simulink model "MPC_mobile_base"  (R2018b)
settings: Solver=ode4  StartTime=0.0  StopTime=60  FixedStep=T  RelTol=1e-3
values from neighbouring files (symbols this model uses):
  N = 3    [MPC_dyn_N=3arc traj.mat]    (also in MPC_dyn_N=3arc traj_active.mat; MPC_dyn_N=3complex traj.mat; MPC_dyn_N=3complex traj_active.mat; MPC_dyn_N=6arc traj.mat = 6)
  T = 0.5    [MPC_dyn_N=3arc traj.mat]    (also in MPC_dyn_N=3arc traj_active.mat; MPC_dyn_N=3complex traj.mat; MPC_dyn_N=3complex traj_active.mat; MPC_dyn_N=6arc traj.mat)
  xd = [0 0 0 0 0 0.000654498469498 0.0758636207458 4.96526307585e-05 0.00261799387799 0.227590374774 0.000446873251435 0.00589048622548 ... (153 elements, 3x51)]    [MPC_dyn_N=3arc traj.mat]    (also in MPC_dyn_N=3arc traj_active.mat; MPC_dyn_N=3complex traj.mat = [0 0 0 0.25 0 0 0.5 0 2.44929359829e-17 0.75 -0.024302237621; MPC_dyn_N=3complex traj_active.mat = [0 0 0 0.25 0 0 0.5 0 2.44929359829e-17 0.75 -0.024302237621; MPC_dyn_N=6arc traj.mat)
undefined symbols (not defined in the file or in its folder): DiscIntNeverNeededParam
libraries: simulink x3, templibrary x1
settings Model: Creator=RaffaelePC  LastModifiedBy=Francesco Gennari
settings DebuggingCC: UnderSpecifiedDimensionMsg=warning

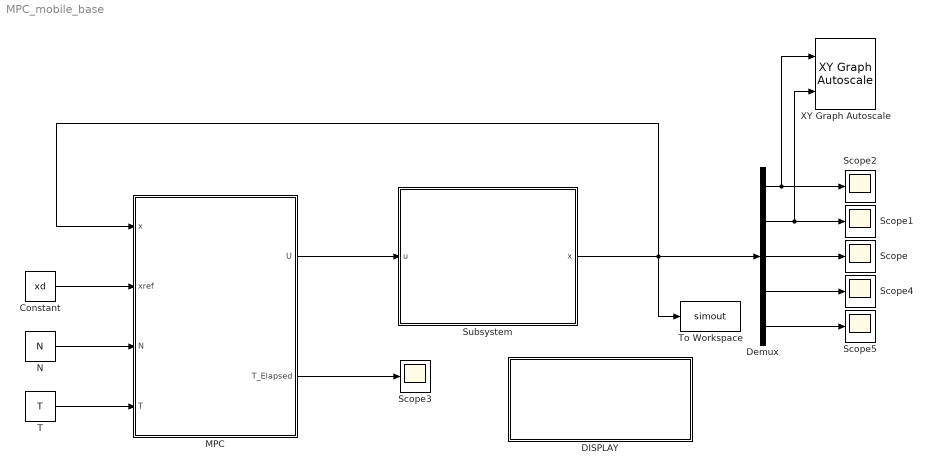
== system MPC_mobile_base ==
  Constant : Constant  Value=xd
  DISPLAY : Subsystem
  Demux : Demux  Outputs=5
  MPC : Subsystem
      mask Display: fprintf('MPC CONTROLLER')
  N : Constant  Value=N
  Scope{,1..5} (6 alike) : Scope
  Subsystem : Subsystem
      mask Display: disp('{\bf\fontsize{10}DYNAMIC SYSTEM}', 'texmode','on');
  T : Constant  Value=T
  To Workspace : ToWorkspace  VariableName=simout  SaveFormat=Timeseries  SampleTime=-1
  XY Graph Autoscale : templibrary/XY Graph  Autoscale  xmin=-1  xmax=1  ymin=-1  ymax=1  st=-1
  wires:
  MPC/1(U) -> Subsystem/1(u)
  N/1 -> MPC/3(N)
  T/1 -> MPC/4(T)
  Constant/1 -> MPC/2(xref)
  Subsystem/1(x) -> To Workspace/1, MPC/1(x), Demux/1
  Demux/3 -> Scope/1
  Demux/1 -> XY Graph Autoscale/1, Scope2/1
  Demux/2 -> XY Graph Autoscale/2, Scope1/1
  MPC/2(T_Elapsed) -> Scope3/1
  Demux/5 -> Scope5/1
  Demux/4 -> Scope4/1

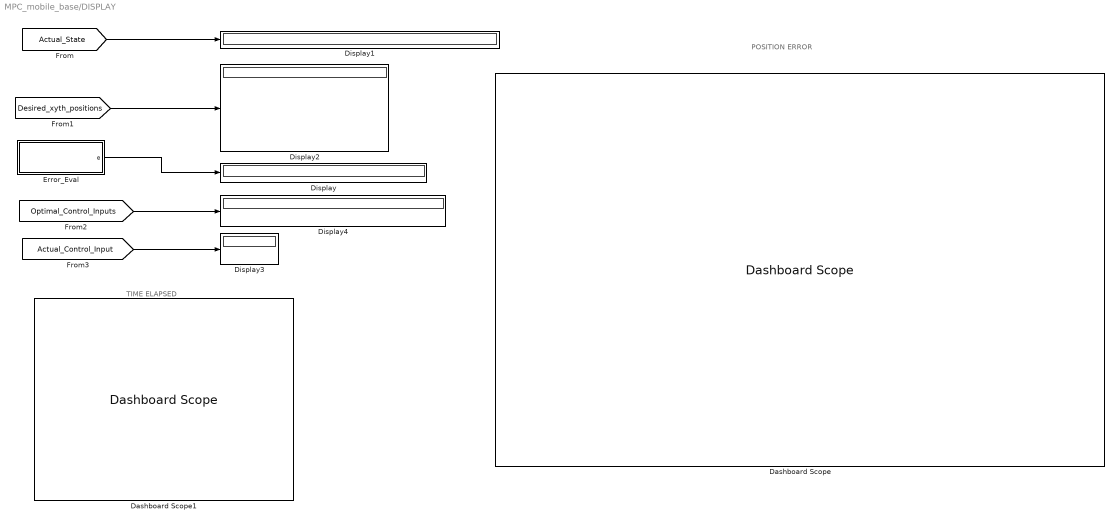
== system MPC_mobile_base/DISPLAY ==
  note: POSITION ERROR
  note: TIME ELAPSED
  Dashboard Scope : DashboardScope  WebBlockId=507  Ymin=-0.5  Ymax=0.5
  Dashboard Scope1 : DashboardScope  WebBlockId=516  Ymin=0  Ymax=1
  Display{,1..4} (5 alike) : Display
  "Error_Eval " : Subsystem
  wires:
  [Optimal_Control_Inputs] -> Display4/1
  [Desired_xyth_positions] -> Display2/1
  [Actual_Control_Input] -> Display3/1
  [Actual_State] -> Display1/1
  "Error_Eval "/1(e) -> Display/1

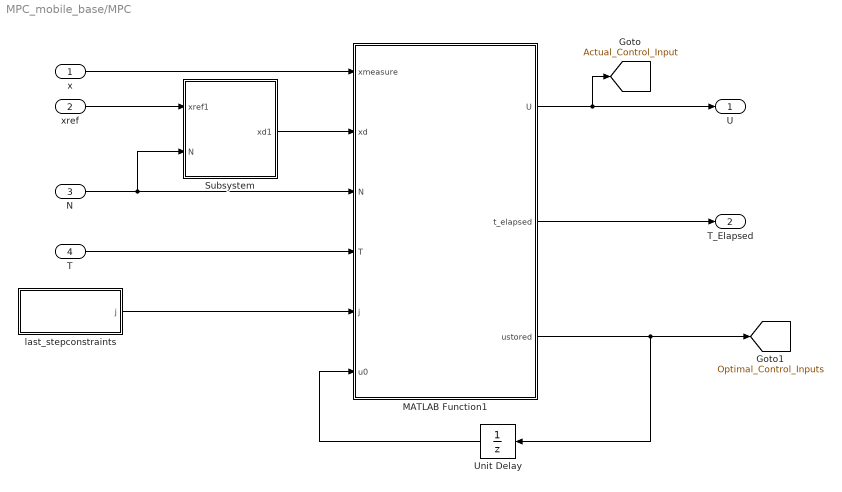
== system MPC_mobile_base/MPC ==
  x : Inport
  xref : Inport  Port=2
  N : Inport  Port=3
  T : Inport  Port=4
  MATLAB Function1 : MATLAB Function  TreatAsAtomicUnit=on
  Subsystem : Subsystem
  Unit Delay : UnitDelay  InitialCondition=zeros(2,N)  SampleTime=-1
  last_stepconstraints : Subsystem
  U : Outport
  T_Elapsed : Outport  Port=2
  tag scope: Actual_Control_Input=global, Optimal_Control_Inputs=global
  wires:
  Subsystem/1(xd1) -> MATLAB Function1/2(xd)
  MATLAB Function1/1(U) -> [Actual_Control_Input], U/1
  MATLAB Function1/3(ustored) -> Unit Delay/1, [Optimal_Control_Inputs]
  Unit Delay/1 -> MATLAB Function1/6(u0)
  xref/1 -> Subsystem/1(xref1)
  x/1 -> MATLAB Function1/1(xmeasure)
  N/1 -> Subsystem/2(N), MATLAB Function1/3(N)
  T/1 -> MATLAB Function1/4(T)
  last_stepconstraints/1(j) -> MATLAB Function1/5(j)
  MATLAB Function1/2(t_elapsed) -> T_Elapsed/1

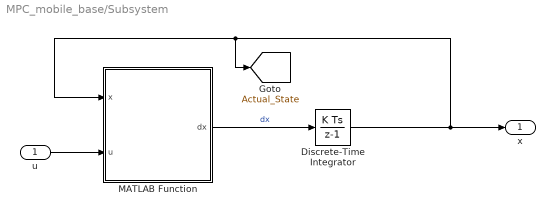
== system MPC_mobile_base/Subsystem ==
  u : Inport
  Discrete-Time Integrator : DiscreteIntegrator  InitialCondition=[xd(:,1).' 0 0]'  SampleTime=-1  ICPrevOutput=DiscIntNeverNeededParam  ICPrevScaledInput=DiscIntNeverNeededParam
  MATLAB Function : MATLAB Function  TreatAsAtomicUnit=on
  x : Outport
  tag scope: Actual_State=global
  wires:
  u/1 -> MATLAB Function/2(u)
  MATLAB Function/1(dx) -> Discrete-Time Integrator/1  "dx"
  Discrete-Time Integrator/1 -> [Actual_State], MATLAB Function/1(x), x/1

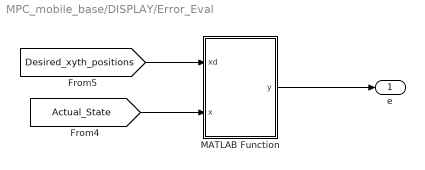
== system MPC_mobile_base/DISPLAY/Error_Eval  ==
  MATLAB Function : MATLAB Function  TreatAsAtomicUnit=on
  e : Outport
  wires:
  MATLAB Function/1(y) -> e/1
  [Desired_xyth_positions] -> MATLAB Function/1(xd)
  [Actual_State] -> MATLAB Function/2(x)

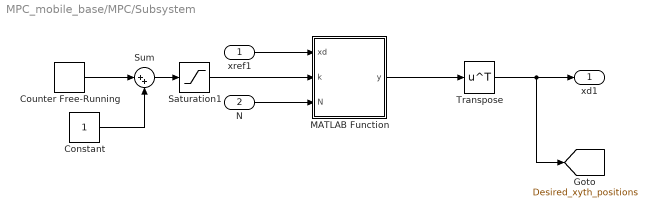
== system MPC_mobile_base/MPC/Subsystem ==
  xref1 : Inport
  N : Inport  Port=2
  Constant : Constant
  Counter Free-Running : simulink/Sources/Counter Free-Running  NumBits=12  tsamp=-1
  MATLAB Function : MATLAB Function  TreatAsAtomicUnit=on
  Saturation1 : Saturate  UpperLimit=size(xd,2)
  Sum : Sum  Inputs=|++
  Transpose : Math  Operator=transpose  SaturateOnIntegerOverflow=on
  xd1 : Outport
  tag scope: Desired_xyth_positions=global
  wires:
  Transpose/1 -> [Desired_xyth_positions], xd1/1
  MATLAB Function/1(y) -> Transpose/1
  N/1 -> MATLAB Function/3(N)
  xref1/1 -> MATLAB Function/1(xd)
  Constant/1 -> Sum/2
  Counter Free-Running/1 -> Sum/1
  Sum/1 -> Saturation1/1
  Saturation1/1 -> MATLAB Function/2(k)

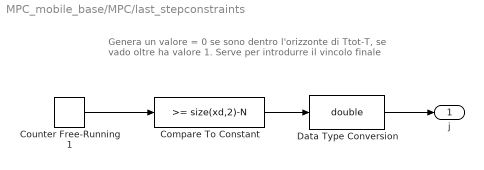
== system MPC_mobile_base/MPC/last_stepconstraints ==
  note: Genera un valore = 0 se sono dentro l'orizzonte di Ttot-T, se vado oltre ha valore 1. Serve per introdurre il vincolo finale
  Compare To Constant : simulink/Logic and Bit Operations/Compare To Constant  relop=>=  const=size(xd,2)-N  OutDataTypeStr=boolean
  Counter Free-Running1 : simulink/Sources/Counter Free-Running  NumBits=12  tsamp=-1
  Data Type Conversion : DataTypeConversion  OutDataTypeStr=double
  j : Outport
  wires:
  Compare To Constant/1 -> Data Type Conversion/1
  Counter Free-Running1/1 -> Compare To Constant/1
  Data Type Conversion/1 -> j/1

== matlab function MPC_mobile_base/MPC/Subsystem/MATLAB Function ==
  settings: updateMethod=DISCRETE  sampleTime=T
  data: xd input; y output size=[3 N+1]; k input; N input
function y  = fcn(xd,k,N)

if size(xd,2)-k>=N
h=xd(:,k:k+N);
y=h;
else
h=[xd(:,k:end) xd(:,end)*ones(1,N-(size(xd,2)-k))];
y = h;
end

== matlab function MPC_mobile_base/MPC/MATLAB Function1 ==
  settings: updateMethod=DISCRETE  sampleTime=T
  data: xmeasure input size=5; U output size=[2 1]; t_elapsed output double size=[1]; xd input; N input; T input; j input; u0 input size=[2 N]; ustored output double size=[2 N] [..20]
function [U,t_elapsed,ustored] = MPC(xmeasure,xd,N,T,j,u0)
coder.extrinsic('tic')
coder.extrinsic('toc')
coder.extrinsic('MPCSOLVER');

t_elapsed=0;

t_start=tic;

U=zeros(2,1); u = zeros(2,N);
xs=xd;
    
u0 = [u0(:,2:size(u0,2)) u0(:,size(u0,2))];

    %% dati solutore


% options = optimset('Display','off',...
%                 'TolFun', 1e-6,...
%                 'MaxIter', 10000,...
%                 'Algorithm', 'active-set',...
%                 'FinDiffType', 'forward',...
%                 'RelLineSrchBnd', [],...
%                 'RelLineSrchBndDuration', 1,...
%                 'TolConSQP', 1e-6);

%% MPC ALGORITHM 

x0=xmeasure';
t0 =0;

if size(xd,1)<N
    U=u0(:,1);
    ustored=u0(:,1:end);
    
else
    
   

    [u_new, V] = MPCSOLVER(N, t0, x0, u0, T, xs, xd,j);

%   [u_new, V] = solveOptimalControlProblem ...
%         (@runningcosts, @terminalcosts, @constraints, @terminalconstraints, ...
%         @linearconstraints, @system, N, t0, x0, u0, T, xs, xd);
     
    ustored=u_new;

    U(1)=u_new(1,1);
    U(2)=u_new(2,1);
    
    
t_elapsed=toc(t_start);

end 

end

== matlab function MPC_mobile_base/DISPLAY/Error_Eval /MATLAB Function ==
  settings: updateMethod=DISCRETE  sampleTime=T
  data: xd input; y output size=[3 1]; x input
function y = fcn(xd,x)

h = [xd(1,1)-x(1);xd(1,2)-x(2);xd(1,3)-x(3)];
y=h;

== matlab function MPC_mobile_base/Subsystem/MATLAB Function ==
  settings: updateMethod=DISCRETE  sampleTime=T
  data: x input; dx output; u input size=[2 1]
function dx = sys_dynamics(x,u)

[A,F,D] = matriceseval(x);
       
 dx=A*x + F*u + D;

end
